simulink model "Gesamtmodell_2015b"  (R2015b)
settings: Solver=ode3  StartTime=0.0  StopTime=inf  FixedStep=dt  RelTol=1e-3
undefined symbols (not defined in the file or in its folder): Com1, dt, K1, K2, K3, Kpsi, Kx, Ky, none, sigbuilder_block, Tpsi, Tx, Ty
libraries: xpcrtudplib x9, xpcobsoletelib x4, simulink x2, xpcseriallib x1, slrtlib x1
(part 2 of 3)

== matlab function Gesamtmodell_2015b/Regelung/Robotino interface/transmit velocity, unit & direction converter ==
  settings: sampleTime=2*dtpc
  data: direction_motor0_out output; velocity_motor0_out output; direction_motor1_out output; velocity_motor1_out output; direction_motor2_out output; velocity_motor2_out output; v_x_in input; v_y_in input; v_theta_in input
%%%%%%%%%%%%%%%%%%%%%%%%%%%%%%%%%%%%%%%%%%%%%%%%%%%%%%%%%%%%%%%%%%%%%%%%%%%
% conversion from positive and/or negative longitudinal, lateral and      %
% rotational velocities (in milimeters per second) to three separate      %
% positive motor velocities (resolution: 1Byte) and their rotation        %
% direction                                                               %
%                                                                         %
% inputs:  v_x_in (longitudinal velocity in milimeters per second),       %
%          v_y_in (lateral velocity in milimeters per second),            %
%          v_theta_in (rotational velocity in milimeters per second)      %
% outputs: direction_motor0_out (rotating direction of motor0             %
%          (0 := counter-clockwise; 2 := clockwise)),                     %
%          velocity_motor0_out (from 0 to 255),                           %
%          direction_motor1_out (rotating direction of motor1             %
%          (0 := counter-clockwise; 2 := clockwise)),                     %
%          velocity_motor1_out (from 0 to 255),                           %
%          direction_motor2_out (rotating direction of motor2             %
%          (0 := counter-clockwise; 2 := clockwise)),                     %
%          velocity_motor2_out (from 0 to 255)                            %
%%%%%%%%%%%%%%%%%%%%%%%%%%%%%%%%%%%%%%%%%%%%%%%%%%%%%%%%%%%%%%%%%%%%%%%%%%%
function [direction_motor0_out, velocity_motor0_out, ...
          direction_motor1_out, velocity_motor1_out, ...
          direction_motor2_out, velocity_motor2_out] ...
                                          = fcn(v_x_in, v_y_in, v_theta_in)
%%%%%%%%%%%%%%%%%%%%%%%%%%%%%%%%%%%%%%%%%%%%%%%%%%%%%%%%%%%%%%%%%%%%%%
% conversion from longitudinal, lateral & rotational velocity to the %
% three separate motor velocities                                    %
%%%%%%%%%%%%%%%%%%%%%%%%%%%%%%%%%%%%%%%%%%%%%%%%%%%%%%%%%%%%%%%%%%%%%%
v0 = (-v_x_in * cosd(30)) + ( v_y_in * cosd(60)) + (v_theta_in * 135);
v1 =                      + (-v_y_in)            + (v_theta_in * 135);
v2 = ( v_x_in * cosd(30)) + ( v_y_in * cosd(60)) + (v_theta_in * 135);

%%%%%%%%%%%%%%%%%%%%%%%%%%%%%%%%%%%%%%%%%%%%%%%%%%%%%%%%%%%%%%%%%%%%%
% conversion of the separate motor velocities from millimeters to a %
% value between -255 and 255                                        %
%%%%%%%%%%%%%%%%%%%%%%%%%%%%%%%%%%%%%%%%%%%%%%%%%%%%%%%%%%%%%%%%%%%%%
f = 1 / 7.02;
v0 = v0 * f;
v1 = v1 * f;
v2 = v2 * f;

%%%%%%%%%%%%%%%%%%%%%%%%%%%%%%%%%%%%%%%%%%%%%%%%%%%%%%%%%%%%%%%%%%%%
% division of motor velocities into absolute velocity and rotating %
% direction                                                        %
%%%%%%%%%%%%%%%%%%%%%%%%%%%%%%%%%%%%%%%%%%%%%%%%%%%%%%%%%%%%%%%%%%%%
if v0 < 0
    direction_motor0_out =  0;
    velocity_motor0_out  = -v0;
else
    direction_motor0_out = 2;
    velocity_motor0_out  = v0;
end

if v1 < 0
    direction_motor1_out =  0;
    velocity_motor1_out  = -v1;
else
    direction_motor1_out = 2;
    velocity_motor1_out  = v1;
end

if v2 < 0
    direction_motor2_out =  0;
    velocity_motor2_out  = -v2;
else
    direction_motor2_out = 2;
    velocity_motor2_out  = v2;
end

== matlab function Gesamtmodell_2015b/Regelung/Robotino interface/serial communication/protocol adder & optional velocity adaption ==
  settings: sampleTime=2*dtpc
  data: dir input; vel input; direction_motor0_in input; velocity_motor0_in input; direction_motor1_in input; velocity_motor1_in input; direction_motor2_in input; velocity_motor2_in input; stop_in input; message output
%%%%%%%%%%%%%%%%%%%%%%%%%%%%%%%%%%%%%%%%%%%%%%%%%%%%%%%%%%%%%%%%%%%%%%%%%%%
% parameterising the 'PC104 to I/O-Board message' for serial line         %
% communication with control commands for the robotino motors             %
%                                                                         %
% optional: velocity adaption as soon as at least one motor is near the   %
%           speed limit                                                   %
%                                                                         %
% inputs: rotating directions and velocities of the three motors          %
% output: vector containing the 'PC104 to I/O-Board message' for serial   %
%         line communication                                              %
%%%%%%%%%%%%%%%%%%%%%%%%%%%%%%%%%%%%%%%%%%%%%%%%%%%%%%%%%%%%%%%%%%%%%%%%%%%
function message = fcn(dir, vel, direction_motor0_in, velocity_motor0_in, ...
                       direction_motor1_in, velocity_motor1_in, ...
                       direction_motor2_in, velocity_motor2_in, stop_in)
%%%%%%%%%%%%%%%%%%%%%%%%%%%%%%
% optional velocity adaption %
%%%%%%%%%%%%%%%%%%%%%%%%%%%%%%
vmax = 175;                                               % v_motor_dez_max

if velocity_motor0_in > vmax
    velocity_motor0_tf = velocity_motor0_in;
    
    velocity_motor0_in = vmax;
    velocity_motor1_in = vmax * velocity_motor1_in / velocity_motor0_tf;
    velocity_motor2_in = vmax * velocity_motor2_in / velocity_motor0_tf;
end

if velocity_motor1_in > vmax
    velocity_motor1_tf = velocity_motor1_in;
    
    velocity_motor0_in = vmax * velocity_motor0_in / velocity_motor1_tf;
    velocity_motor1_in = vmax;
    velocity_motor2_in = vmax * velocity_motor2_in / velocity_motor1_tf;
end

if velocity_motor2_in > vmax
    velocity_motor2_tf = velocity_motor2_in;
    
    velocity_motor0_in = vmax * velocity_motor0_in / velocity_motor2_tf;
    velocity_motor1_in = vmax * velocity_motor1_in / velocity_motor2_tf;
    velocity_motor2_in = vmax;
end
%%%%%%%%%%%%%%%%%%%%%%%%%%%%%%%%%%%%%%%%%%%%%%%%%%%%%%%%%%%%%%%%%%%%%%
% vector containing the 'PC104 to I/O-Board message' for serial line %
% communication                                                      %
%%%%%%%%%%%%%%%%%%%%%%%%%%%%%%%%%%%%%%%%%%%%%%%%%%%%%%%%%%%%%%%%%%%%%%
message = [47, abs('REC'), 5, min(stop_in), direction_motor0_in, ...
           velocity_motor0_in, zeros(1, 4), 255, 255, 255, ...
           min(stop_in), direction_motor1_in, velocity_motor1_in, ...
           zeros(1, 4), 255, 255, 255, min(stop_in), ...
           direction_motor2_in, velocity_motor2_in, zeros(1, 4), 255, ...
           255, 255, 1, dir, vel, zeros(1, 4), 255, 255, 255, abs('rec')].';

== matlab function Gesamtmodell_2015b/Regelung/Receiver/UDP interface/stop signals ==
  data: rob_number input; udp_in input; enable_out output
%%%%%%%%%%%%%%%%%%%%%%%%%%%%%%%%%%%%%%%%%%%%%%%%%%%%%%%%%%%%%%%%%%%%%%%%%%%
% Leads the enable command through. The enable command turns the Robotino %
% inputs to selectable form.                                              %
%                                                                         %
% input: udp_in (vector of 56 elements containing the data sent by the    %
%                camera-model)                                            %
% outputs: enable_out (1 = inputs are in selectable form;                 %
%                      0 = inputs are set to 0)                           %
%          udp_out (vector of 56 elements containing the data sent by the %
%                   camera-model)                                         %
%%%%%%%%%%%%%%%%%%%%%%%%%%%%%%%%%%%%%%%%%%%%%%%%%%%%%%%%%%%%%%%%%%%%%%%%%%%
function enable_out  = fcn(rob_number, udp_in)
enable_out = [0, 0];
if (udp_in(rob_number * 3 - 2) <= 0) && ...
   (udp_in(rob_number * 3 - 1) <= 0) && (udp_in(rob_number * 3) <= 0)
    enable_out(1) = 0;
else
    enable_out(1) = 1;
end
enable_out(2) = udp_in(28);

== matlab function Gesamtmodell_2015b/Regelung/Robotino interface/serial communication/error filter & protocol disassembler ==
  settings: sampleTime=dtpc/2
  data: response input; error_free_resp_in input; direction_motor0_out output; velocity_motor0_out output; direction_motor1_out output; velocity_motor1_out output; direction_motor2_out output; velocity_motor2_out output; distance_measuring_sensors_out output; di03_bump_out output; bumper_out output; error_free_resp_out output
%%%%%%%%%%%%%%%%%%%%%%%%%%%%%%%%%%%%%%%%%%%%%%%%%%%%%%%%%%%%%%%%%%%%%%%%%%%
% Error check of the 'I/O-Board to PC104 message' and filtering of this   %
% defective response: Substitute defective message by the last error free %
% message.                                                                %
% Saving of the rotating direction, velocity, shaft position and running  %
% time of the three motors. Combining all shaft positions in a vector.    %
% Combining all running times in a vector.                                %
% Saving of the three bumper bytes indicating a collision in a vector.    %
% Saving the values of the nine distance measuring IR-sensors in a vector.%
%                                                                         %
% inputs: response (actual 'I/O-Board to PC104 message')(vector 102       %
%                   elements)                                             %
%         error_free_resp_in (last error free 'I/O-Board to PC104         %
%                             message')                                   %
% outputs: directions and velocities of the three motors                  %
%          motor_positions_out (shaft positions of the three motors)      %
%                              (vector 12 elements)                       %
%          time_bytes_out (running times of the three motors)             %
%                         (vector 9 elements)                             %
%          distance_measuring_sensors_out (values of the nine IR-sensors) %
%                                         (vector 9 elements)             %
%          bumper_out (vector 3 elements)                                 %
%          error_free_resp_out (error free 'I/O-Board to PC104 message')  %
%                              (vector 102 elements)                      %
%%%%%%%%%%%%%%%%%%%%%%%%%%%%%%%%%%%%%%%%%%%%%%%%%%%%%%%%%%%%%%%%%%%%%%%%%%%
function [direction_motor0_out, velocity_motor0_out, ...
          direction_motor1_out, velocity_motor1_out, ...
          direction_motor2_out, velocity_motor2_out, ...
          distance_measuring_sensors_out, di03_bump_out, bumper_out, ...
          error_free_resp_out] = fcn(response, error_free_resp_in)
%           motor_positions_out, time_bytes_out, ...)
      
%%%%%%%%%%%%%%%%%%%%%%%%%%%%%%%%%%%%%%%%%%%%%%%%%%%%%
% filtering defective 'I/O-Board to PC104 messages' %
%%%%%%%%%%%%%%%%%%%%%%%%%%%%%%%%%%%%%%%%%%%%%%%%%%%%%
if (response(1) == 101) && (response(2) == 82) && (response(3) == 69) ...
   && (response(4) == 67) && (response(100) == 114) ...        % if the ...
   && (response(101) == 101) && (response(102) == 99)  % counter (101), ...
                        % the start (REC) and stop (rec) bytes are true ...
    error_free_resp_out = response;     % save the actual 'I/O-Board to ...
                                                           % PC104 message'
else                                                        % otherwise ...
    error_free_resp_out = error_free_resp_in;     % save the last error ...
                                        % free 'I/O-Board to PC104 message'
end

%%%%%%%%%%%%%%%%%%%%%%%%%%%%%%%%%%%%%%%%%%%%%%%%%%%%%%%%%%%%%%%%%%%%%%%%%%
% save rotating direction, velocity, shaft position and the running time %
% of motor0                                                              %
%%%%%%%%%%%%%%%%%%%%%%%%%%%%%%%%%%%%%%%%%%%%%%%%%%%%%%%%%%%%%%%%%%%%%%%%%%
direction_motor0_out  = error_free_resp_out(26);
velocity_motor0_out   = error_free_resp_out(27);
% position_motor0_byte1 = error_free_resp_out(28);
% position_motor0_byte2 = error_free_resp_out(29);
% position_motor0_byte3 = error_free_resp_out(30);
% position_motor0_byte4 = error_free_resp_out(31);
% time_motor0_byte1     = error_free_resp_out(34);
% time_motor0_byte2     = error_free_resp_out(35);
% time_motor0_byte3     = error_free_resp_out(36);

%%%%%%%%%%%%%%%%%%%%%%%%%%%%%%%%%%%%%%%%%%%%%%%%%%%%%%%%%%%%%%%%%%%%%%%%%%
% save rotating direction, velocity, shaft position and the running time %
% of motor1                                                              %
%%%%%%%%%%%%%%%%%%%%%%%%%%%%%%%%%%%%%%%%%%%%%%%%%%%%%%%%%%%%%%%%%%%%%%%%%%
direction_motor1_out  = error_free_resp_out(47);
velocity_motor1_out   = error_free_resp_out(48);
% position_motor1_byte1 = error_free_resp_out(49);
% position_motor1_byte2 = error_free_resp_out(50);
% position_motor1_byte3 = error_free_resp_out(51);
% position_motor1_byte4 = error_free_resp_out(52);
% time_motor1_byte1     = error_free_resp_out(55);
% time_motor1_byte2     = error_free_resp_out(56);
% time_motor1_byte3     = error_free_resp_out(57);

%%%%%%%%%%%%%%%%%%%%%%%%%%%%%%%%%%%%%%%%%%%%%%%%%%%%%%%%%%%%%%%%%%%%%%%%%%
% save rotating direction, velocity, shaft position and the running time %
% of motor2                                                              %
%%%%%%%%%%%%%%%%%%%%%%%%%%%%%%%%%%%%%%%%%%%%%%%%%%%%%%%%%%%%%%%%%%%%%%%%%%
direction_motor2_out  = error_free_resp_out(68);
velocity_motor2_out   = error_free_resp_out(69);
% position_motor2_byte1 = error_free_resp_out(70);
% position_motor2_byte2 = error_free_resp_out(71);
% position_motor2_byte3 = error_free_resp_out(72);
% position_motor2_byte4 = error_free_resp_out(73);
% time_motor2_byte1     = error_free_resp_out(76);
% time_motor2_byte2     = error_free_resp_out(77);
% time_motor2_byte3     = error_free_resp_out(78);

%%%%%%%%%%%%%%%%%%%%%%%%%%%%%%%%%%%%%%%%%%%
% save the three bumper bytes in a vector %
%%%%%%%%%%%%%%%%%%%%%%%%%%%%%%%%%%%%%%%%%%%
bumper_out = [error_free_resp_out(32), error_free_resp_out(53), ...
              error_free_resp_out(74)]';
          
%%%%%%%%%%%%%%%%%%%%%%%%%%%%%%%%%%%%%%%%%%%%%%%%%%%%%%%%%%%%%%%%%%%%%%
% save the values of the nine distance measuring sensors in a vector %
%%%%%%%%%%%%%%%%%%%%%%%%%%%%%%%%%%%%%%%%%%%%%%%%%%%%%%%%%%%%%%%%%%%%%%
distance_measuring_sensors_out = [error_free_resp_out(60), ...
                    error_free_resp_out(59), error_free_resp_out(44), ...
                    error_free_resp_out(39), error_free_resp_out(38), ...
                    error_free_resp_out(17), error_free_resp_out(18), ...
                    error_free_resp_out(23), error_free_resp_out(65)];
                
%%%%%%%%%%%%%%%%%%%%%%%%%%%%%%%%%%%%%%%%%%%%%%%%%%%%%%%%
% save positions of the three motor shafts in a vector %
%%%%%%%%%%%%%%%%%%%%%%%%%%%%%%%%%%%%%%%%%%%%%%%%%%%%%%%%
% motor_positions_out = [position_motor0_byte1, position_motor0_byte2, ...
%                        position_motor0_byte3, position_motor0_byte4, ...
%                        position_motor1_byte1, position_motor1_byte2, ...
%                        position_motor1_byte3, position_motor1_byte4, ...
%                        position_motor2_byte1, position_motor2_byte2, ...
%                        position_motor2_byte3, position_motor2_byte4];

%%%%%%%%%%%%%%%%%%%%%%%%%%%%%%%%%%%%%%%%%%%%%%%%%%%%%%%%%%
% save the running times of the three motors in a vector %
%%%%%%%%%%%%%%%%%%%%%%%%%%%%%%%%%%%%%%%%%%%%%%%%%%%%%%%%%%
% time_bytes_out = [time_motor0_byte1, time_motor0_byte2, ...
%                   time_motor0_byte3, time_motor1_byte1, ...
%                   time_motor1_byte2, time_motor1_byte3, ...
%                   time_motor2_byte1, time_motor2_byte2, time_motor2_byte3];

%%%%%%%%%%%%%%%%%%%%%%%%%%%%%%%%%%%%%%
% save values of digital input 0 - 3 %
%%%%%%%%%%%%%%%%%%%%%%%%%%%%%%%%%%%%%%
di03_bump_out = error_free_resp_out(32);

== matlab function Gesamtmodell_2015b/Regelung/Robotino interface/receive direction, unit & velocity converter ==
  settings: sampleTime=dtpc/2
  data: number_of_robot input; direction_motor0_in input; v_x_out output; velocity_motor0_in input; direction_motor1_in input; velocity_motor1_in input; direction_motor2_in input; velocity_motor2_in input; v_y_out output; v_theta_out output
%%%%%%%%%%%%%%%%%%%%%%%%%%%%%%%%%%%%%%%%%%%%%%%%%%%%%%%%%%%%%%%%%%%%%%%%%%%
% assembly of the three separate positive motor velocities (resolution:   %
% 1Byte) and their rotation direction to positive and/or negative         %
% longitudinal, lateral & rotational velocities (in milimeters per        %
% second)                                                                 %
%                                                                         %
% inputs:  direction_motor0_in (rotating direction of motor0              %
%          (129 := counter-clockwise; 128 := clockwise)),                 %
%          velocity_motor0_in (from 0 to 255),                            %
%          direction_motor1_in (rotating direction of motor1              %
%          (0 := counter-clockwise; 1 := clockwise)),                     %
%          velocity_motor1_in (from 0 to 255),                            %
%          direction_motor2_in (rotating direction of motor2              %
%          (0 := counter-clockwise; 1 := clockwise)),                     %
%          velocity_motor2_in (from 0 to 255)                             %
% outputs: v_x_out (longitudinal velocity (in milimeters per second)),    %
%          v_y_out (lateral velocity (in milimeters per second)),         %
%          v_theta_out (rotational velocity (in milimeters per second))   %
%%%%%%%%%%%%%%%%%%%%%%%%%%%%%%%%%%%%%%%%%%%%%%%%%%%%%%%%%%%%%%%%%%%%%%%%%%%
function [v_x_out, v_y_out, v_theta_out] ...
    = fcn(number_of_robot, direction_motor0_in, velocity_motor0_in, direction_motor1_in, ...
          velocity_motor1_in, direction_motor2_in, velocity_motor2_in)
%%%%%%%%%%%%%%%%%%%%%%%%%%%%%%%%%%%%%%%%%%%%%%%%%%%%%%%%%%%%%%%%%
% assembly of absolute motor velocity and rotating direction to %
% longitudinal, lateral & rotational velocity for every motor   %
%%%%%%%%%%%%%%%%%%%%%%%%%%%%%%%%%%%%%%%%%%%%%%%%%%%%%%%%%%%%%%%%%


% the direction bit for the motor 0 of robotino 3 is located at a different position
if number_of_robot == 3
    cmp = 1;
else
    cmp = 129;
end
    

if direction_motor0_in < cmp
    v0 = -velocity_motor0_in;
else
    v0 =  velocity_motor0_in;
end

if direction_motor1_in < 1
    v1 = -velocity_motor1_in;
else
    v1 =  velocity_motor1_in;
end

if direction_motor2_in < 1
    v2 = -velocity_motor2_in;
else
    v2 =  velocity_motor2_in;
end

%%%%%%%%%%%%%%%%%%%%%%%%%%%%%%%%%%%%%%%%%%%%%%%%%%%%%%%%%%%%%%%%%%%%%%%%%
% conversion of the separate motor velocities from a value between -255 %
% and 255 to millimeters                                                %
%%%%%%%%%%%%%%%%%%%%%%%%%%%%%%%%%%%%%%%%%%%%%%%%%%%%%%%%%%%%%%%%%%%%%%%%%
f_rcv = 7.02;
v0    = v0 * f_rcv;
v1    = v1 * f_rcv;
v2    = v2 * f_rcv;

%%%%%%%%%%%%%%%%%%%%%%%%%%%%%%%%%%%%%%%%%%%%%%%%%%%%%%%%%%%%%%%%%%%%
% conversion from three separate motor velocities to longitudinal, %
% lateral & rotational velocity                                    %
%%%%%%%%%%%%%%%%%%%%%%%%%%%%%%%%%%%%%%%%%%%%%%%%%%%%%%%%%%%%%%%%%%%%
v_x_out     = (v2 - v0) / (2 * cosd(30));                         % in mm/s
v_y_out     = (v0 - 2 * v1 + v2) / 3;                             % in mm/s
v_theta_out = (v0 + v1 + v2) / (3 * 135);                        % in rad/s

== matlab function Gesamtmodell_2015b/Regelung/Receiver/autoRobID ==
  data: udpIn input; pX output; pY output; psi output; enable output; robID input
function [pX, pY, psi, enable] = autoRobID(udpIn, robID)
enable  = 1;
pX      = 0;
pY      = 0;
psi     = 0;

if robID == 1
    pX      = udpIn(1);
    pY      = udpIn(2);
    psi     = udpIn(3);
elseif robID == 2
    pX      = udpIn(4);
    pY      = udpIn(5);
    psi     = udpIn(6);
elseif robID == 3
    pX      = udpIn(7);
    pY      = udpIn(8);
    psi     = udpIn(9);
elseif robID == 4
    pX      = udpIn(10);
    pY      = udpIn(11);
    psi     = udpIn(12);
end

if (pX == 0) && (pY == 0)
    enable = 0;
end

== matlab function Gesamtmodell_2015b/Regelung/Robotino interface/serial communication/stop by bumper ==
  settings: sampleTime=2*dtpc
  data: stop_out output; bumper input; stop_flag_in input; stop_flag_out output
%%%%%%%%%%%%%%%%%%%%%%%%%%%%%%%%%%%%%%%%%%%%%%%%%%%%%%%%%%%%%%%%%%%%%%%%%%%
% Recognition of collisions and creating of variables indicating and      %
% marking a collision                                                     %
%                                                                         %
% inputs: bumper (vector of the three bumper bytes)                       %
%         stop_flag_in (As long as no collision has occured,              %
%                       'stop_flag_in' contains the last bumper vector    %
%                       indicating no collision.                          %
%                       If a collision has occured, 'stop_flag_in'        %
%                       contains the last bumper vector indicating a      %
%                       collision until the simulation stops.)            %
% outputs: stop_out (indicates a collision: 1 = no collision;             %
%                                           0 = collision)                %
%          stop_flag_out (gets the actual bumper vector unless 'bumper'   %
%                         indicates no collision and 'stop_flag_in'       %
%                         indicates a past collision.)                    %
%%%%%%%%%%%%%%%%%%%%%%%%%%%%%%%%%%%%%%%%%%%%%%%%%%%%%%%%%%%%%%%%%%%%%%%%%%%
function [stop_out, stop_flag_out] = fcn(bumper, stop_flag_in)
if max(bumper) == 31       % as soon as the maximum value of the bumper ...
                              % vector indicates 31 a collision is detected
    stop_out = 0;
    stop_flag_out = bumper;
elseif max(stop_flag_in) == 31 % if the maximum value of 'stop_flag_in' ...
                                      % indicates a past collision (31) ...
    stop_out = 0;         % 'stop_out' gets 0 for a further stop of the ...
                                                           % motors and ...
    stop_flag_out = stop_flag_in; % 'stop_flag_out' gets the last bumper...
                                       % vector indicating a past collision
else                                                        % otherwise ...
    stop_out = 1;    % 'stop_out' gets 1 to keep the motors running and ...
    stop_flag_out = bumper; % 'stop_flag_out' gets the actual bumper vector
end

== matlab function Gesamtmodell_2015b/Regelung/Robotino interface/distance converter ==
  settings: sampleTime=dtpc/2
  data: dms_in input; dms_out output
%%%%%%%%%%%%%%%%%%%%%%%%%%%%%%%%%%%%%%%%%%%%%%%%%%%%%%%%%%%%%%%%%%%%%%%%%%%
% conversion of the nine distance measuring sensor values (resolution:    %
% 1Byte) to unit milimeters (range: from 40mm to 1500mm) with linear      %
% interpolation                                                           %
%                                                                         %
% input:  vector containing the values of the nine distance measuring     %
%         sensors                                                         %
% output: vector containing the nine values in milimeters                 %
%%%%%%%%%%%%%%%%%%%%%%%%%%%%%%%%%%%%%%%%%%%%%%%%%%%%%%%%%%%%%%%%%%%%%%%%%%%
function dms_out = fcn(dms_in)

y_mm = [40, 45, 50, 60, 75, 100, 125, 150, 175, 200, 250, 300]; % , ...
        %400, 500, 600, 700, 800, 900, 1000, 1100, 1200, 1300, 1500];
    
x_sensor = [255, 249.7733813, 228.6082474, 193.6871795, ...
            152.0044843, 113.7266187, 92.42268041, ...
            76.36407767, 65.19289827, 55.1025641, ...
            43.06299213, 34.97068404]; % , 24.37410072, ...
            % 16.3381295, 11.62589928, 8.661870504, ...
            % 6.316546763, 4.74, 3.65, 2.96, 2.40, ...
            % 2.035971223, 1.539568345];

% x_sensor = round(100 * x_sensor) / 100;

dms_out = interp1(x_sensor, y_mm, dms_in, 'linear');

== matlab function Gesamtmodell_2015b/Regelung/z(x) ==
  data: x1 input; x2 input; x3 input; x4 input; z1 output; z5 output; z2 output; z6 output; x5 input; x6 input; z3 output; z4 output
function [z1,z5,z2,z6,z3,z4]= zustandsTrafo(x1,x2,x3,x4,x5,x6)

z1 = cos(x4) * x1 - sin(x4) * x2;
z2 = sin(x4) * x1 + cos(x4) * x2;
z3 = x3;
z4 = x4;
z5 = x5;
z6 = x6;

== matlab function Gesamtmodell_2015b/Regelung/Robotino interface/light barrier & slider ==
  data: di03_bump_in input; light_barrier output; slider output
function [light_barrier, slider] = fcn(di03_bump_in)
%%%%%%%%%%%%%%%%%%%%%%%%%%%%%%%%%%%%%%%%%%%%%%%%%%%%%%%%%%%%%%%%%%%%%%%%%%%
% di03_bump_in = 0 alternatively 12 ->  no light barrier activation       %
%                                       no slider activation              %
% di03_bump_in = 13                 ->  only light barrier activation     %
% di03_bump_in = 14                 ->  only slider activation            %
% di03_bump_in = 15                 ->  light barrier activation          %
%                                       slider activation                 %
%%%%%%%%%%%%%%%%%%%%%%%%%%%%%%%%%%%%%%%%%%%%%%%%%%%%%%%%%%%%%%%%%%%%%%%%%%%
% function [light_barrier, slider] = fcn(di03_bump_in)
% bin = dec2bin(di03_bump_in);
% if bin(3) == 1
%     light_barrier = 1;
% else
%     light_barrier = 0;
% end
% if bin(4) == 1
%     slider = 1;
% else
%     slider = 0;
% end
if     di03_bump_in == 13
    light_barrier = 1;
    slider        = 0;
elseif di03_bump_in == 14
    light_barrier = 0;
    slider        = 1;
elseif di03_bump_in == 15
    light_barrier = 1;
    slider        = 1;
else
    light_barrier = 0;
    slider        = 0;
end

== stateflow chart Gesamtmodell_2015b/Regelung/Zustandsautomat/FertigunsbereichsLogik ==
  state Warten
    entry: ZielAnfordern = 1;
    exit: ZielAnfordern = 0;
  state Neue_Station_erhalten
  note: => Greifer öffnen
  note: => Warten
  state zuerst_Vorposition_anfahren
    entry: StationsNr = Ziel + 5;
  note: => Greifer schließen
  state Ziel_anfahren
    entry: StationsNr = Ziel;
  state zuerst_Vorposition_anfahren2
    entry: StationsNr = letztesZiel + 5;
  state Station_anfahren
    entry: enable = 1,
    Neue_Planung =1;
  state Station_erreicht
    entry: enable = 1,
    Neue_Planung = 0;
    exit: letztesZiel = StationsNr;
  (default) -> Warten
  Station_erreicht -> Warten [order 3] : [AktionAnZiel == 2]
      |  / {GreiferPose = 0}
  Station_erreicht -> Warten [order 4]
  Station_erreicht -> Warten [order 2] : [AktionAnZiel == 1]
      | / {GreiferPose = 1}
  Warten -> Neue_Station_erhalten : [Ziel ~= letztesZiel]
  Neue_Station_erhalten -> zuerst_Vorposition_anfahren [order 2] : [istEinFach(Ziel) &&  ...
      |  ~istVorpositionDesFachs(Ziel, letztesZiel)]
  Station_erreicht -> Neue_Station_erhalten [order 1] : [StationsNr ~= Ziel]
  Neue_Station_erhalten -> zuerst_Vorposition_anfahren2 [order 1] : [istEinFach(Ziel) &&  ...
      |  ~istVorpositionDesFachs(Ziel, letztesZiel) && istEinFach(letztesZiel)]
  Neue_Station_erhalten -> zuerst_Vorposition_anfahren2 [order 3] : [istEinFach(letztesZiel)]
  Neue_Station_erhalten -> Ziel_anfahren [order 4]
  zuerst_Vorposition_anfahren -> Station_anfahren
  Ziel_anfahren -> Station_anfahren
  zuerst_Vorposition_anfahren2 -> Station_anfahren
  Station_anfahren -> Station_erreicht : [zielPositionErreicht]
  data: ziel function_input double; antwort function_output double; Ziel function_input double; letztesZiel function_input double; antwort function_output double; Ziel input double; AktionAnZiel input double; ZielAnfordern output double =0; letztesZiel local double =0; enable output double =0; GreiferPose output double; zielPositionErreicht input; StationsNr output double =0; Neue_Planung output double
  function antwort = istEinFach(ziel):
    | function antwort = istEinFach(ziel)
    |  
    |     if 0 < mod(ziel, 10) &&  mod(ziel, 10) < 4
    |         antwort = 1;
    |     else
    |         antwort = 0;
    |     end
    | 
    | end
  function antwort = istVorpositionDesFachs(Ziel, letztesZiel):
    | function antwort = istVorpositionDesFachs(Ziel, letztesZiel)
    | 
    |     if (letztesZiel - 5) == Ziel
    |         % Fachnummer + 5 = Nummer der Vorposition
    |         antwort = 1;
    |     else
    |         antwort = 0;
    |     end
    | 
    | end

== matlab function Gesamtmodell_2015b/Regelung/Stellgrößen- beschränkung /Beschraenkung  ==
  data: MaxStellT input; MaxStellR input; x input; X output; Y output; y input; theta input; Theta output
function [X,Y,Theta] = Beschraenkung(MaxStellT,MaxStellR,x,y,theta)

if (x > MaxStellT)
    X = MaxStellT;
elseif  (x < -MaxStellT)
    X = -MaxStellT;
else 
    X = x;
end

if (y > MaxStellT)
    Y = MaxStellT;
elseif  (y < -MaxStellT)
    Y = -MaxStellT;
else
    Y = y;
end

if (theta > MaxStellR)
    Theta = MaxStellR;
elseif  (theta < -MaxStellR)
    Theta = -MaxStellR;
else
    Theta = theta;
end

== matlab function Gesamtmodell_2015b/Regelung/u(x,v)  ==
  data: v1 input; v2 input; v3 input; x1 input; x2 input; x3 input; x4 input; u1 output; u2 output; u3 output; Tx parameter; Ty parameter; Kx parameter; Ky parameter
function [u1, u2, u3]= inputLinearisierung(v1,v2,v3,x1,x2,x3,x4,Tx,Ty,Kx,Ky)


%u1 = (Ty*x1 - Tx*x1 + Ty*v1*cos(x4) + Tx*v2*sin(x4) + Tx*x1*cos(x4)^2 - Ty*x1*cos(x4)^2 - (Tx*x2*sin(2*x4))/2 + (Ty*x2*sin(2*x4))/2 + Tx*Ty*x2*x3)/Ty;
%u2 = -(Ty*x2 - Tx*x2 - Tx*v2*cos(x4) + Ty*v1*sin(x4) + Tx*x2*cos(x4)^2 - Ty*x2*cos(x4)^2 + (Tx*x1*sin(2*x4))/2 - (Ty*x1*sin(2*x4))/2 + Tx*Ty*x1*x3)/Tx;
u1 = (Ty*x1 - Tx*x1 + Tx*x1*cos(x4)^2 - Ty*x1*cos(x4)^2 - (Tx*x2*sin(2*x4))/2 + (Ty*x2*sin(2*x4))/2 + Kx*Ty*v1*cos(x4) + Ky*Tx*v2*sin(x4) + Tx*Ty*x2*x3)/(Kx*Ty);
u2 = -(Ty*x2 - Tx*x2 + Tx*x2*cos(x4)^2 - Ty*x2*cos(x4)^2 + (Tx*x1*sin(2*x4))/2 - (Ty*x1*sin(2*x4))/2 - Ky*Tx*v2*cos(x4) + Kx*Ty*v1*sin(x4) + Tx*Ty*x1*x3)/(Ky*Tx);
u3 = v3;

== matlab function Gesamtmodell_2015b/Regelung/Receiver/x4(psi) ==
  data: psi input; x4 output
function x4 = Winkelkorrektur(psi)

persistent turnCounter firstRun lastAngle

if isempty(firstRun)
    firstRun = 1;
    turnCounter = 0;
    lastAngle = 0;
end

% Kamera gibt uns -pi bis + pi
% Wir wollen 0 bis 2pi
psi = mod(psi+2*pi,2*pi);

% winkel kontinuierlich hoch bzw runterzaehlen
if( (psi < (2*pi)/5) && (lastAngle > ((2*pi) - (2*pi)/5) ) )
    turnCounter = turnCounter + 1;
end

if( (lastAngle < (2*pi)/5) && (psi > ((2*pi) - (2*pi)/5) ) )
    turnCounter = turnCounter - 1;
end

lastAngle = psi;

x4 = psi + turnCounter * 2*pi;

== matlab function Gesamtmodell_2015b/Regelung/Zustandsregler/Winkelentstoerung ==
  data: Ist input; Soll input; Out output



function Out = Winkel(Ist,Soll)

Ist = mod(Ist, 2*pi);      % Normierung des Ist-Winkels auf das Intervall 0° - 360°
Soll = mod(Soll, 2*pi);    % Normierung des Soll-Winkels auf das Intervall 0° - 360°

if (abs(Soll-Ist) <= pi)   % (1)
    
    Out = Soll - Ist;      % (2)
    
else
    
     if (Soll > Ist)                % (3)
        Out = Soll - Ist - 2*pi;    % (4)
     else
         Out = Soll - Ist + 2*pi;   % (5)
     end
end

% Problem: 
% Beim Durchschreiten der Grenze 0°/360° entsteht ein Sprung in
% der Regeldifferenz beim Winkel, der zu einer unkontrollierten Rotation
% des Robotino führt
% 
% Lösung: 
% Impelementierung einer Fallunterscheidung, die die tatsächliche
% Regeldifferenz unter Berücksichtigung der Grenze 0°/360° ausgibt
% 
% Ansatz: 
% Prüfung, ob die vorgegebene Trajektorie über die kritische Grenze
% führt (1). Führt die Trajektorie über die kritische Grenze, ist
% der Betrag der Differenz zwischen Soll- und Istwert > pi.
% 
% Bei unkritischen Trajektorien wird die Regeldifferenz über die Formel (2)
% zurückgegeben.
%
% Bei kritischen Trajektorien muss zuerst unterschieden werden, in welchem
% Drehsinn die kritische Grenze durchschritten wird (3). Bei positivem
% Drehsinn wird die Differenz nach Formel (4) ermittelt, bei negativem
% Drehsinn wird die Differenz nach Formal (5) ermittelt. 
%
% Die Ausgabe der Regeldifferenz erfolgt immer in Richtung und Betrag, bei
% einem positiven Vorzeichen befindet sich die Sollposition in mathematisch
% positivem Drehsinn, bei einem negativen Vorzeichen befindet sie sich in
% mathematisch negativem Drehsinn. Der Betrag gibt die verbleibene
% Winkeldifferenz zur Sollposition an.

== matlab function Gesamtmodell_2015b/Regelung/Zustandsautomat/KoordonatenTafel1 ==
  data: stationsNr input; zielX output; zielY output; zielPsi output; StationsKoordinaten parameter; enable output
function [zielX, zielY, zielPsi, enable] = koordinaten(stationsNr,StationsKoordinaten)

enable = 1;

% Warteposition vorne
if mod(stationsNr, 10) == 0 
    
        % WartePosition 0
        if stationsNr == 0
            %weil Matlab leider nicht von 0 aus zählen kann müssen wir das von
            %Hand abfangen...doofes Matlab
            zielX   = 853;
            zielY   = 2288;
            zielPsi = pi/2;
        else
            zielX   = StationsKoordinaten(1,stationsNr);
            zielY   = StationsKoordinaten(2,stationsNr);
            zielPsi = pi/2;
        end

% Stations-Bucht
elseif 0 < mod(stationsNr, 10) && mod(stationsNr, 10) < 4
    
    zielX   = StationsKoordinaten(1,stationsNr);
    zielY   = StationsKoordinaten(2,stationsNr);
    
    % auf welcher Seite der Station?
    if mod(stationsNr, 20) < 10
        % links
        zielPsi = 0;
    else
        % rechts
        zielPsi = pi;
    end

% Warteposition hinten
elseif mod(stationsNr, 10) == 4
    
    zielX   = StationsKoordinaten(1,stationsNr);
    zielY   = StationsKoordinaten(2,stationsNr);
    zielPsi = pi/2;

% Warteposition mitte
elseif mod(stationsNr, 10) == 5
    
    zielX   = StationsKoordinaten(1,stationsNr);
    zielY   = StationsKoordinaten(2,stationsNr);
    zielPsi = pi/2;

% Vorposition der Bucht
elseif 5 < mod(stationsNr, 10) && mod(stationsNr, 10) < 9
    
    % auf welcher Seite der Station?
    if mod(stationsNr, 20) < 10
        % links
        zielX   = StationsKoordinaten(1,stationsNr-5) - 100;
        zielY   = StationsKoordinaten(2,stationsNr-5);
        zielPsi = 0;
    else
        % rechts
        zielX   = StationsKoordinaten(1,stationsNr-5) + 100;
        zielY   = StationsKoordinaten(2,stationsNr-5);
        zielPsi = pi;
    end

% eine nicht zugeteilte Stationsnummer wird angefordert
else
    % Roboter anhalten
    enable = 0;

    zielX   = 0;
    zielY   = 0;
    zielPsi = 0;
end

== matlab function Gesamtmodell_2015b/Regelung/Zustandsautomat/zielErreicht ==
  data: roboX input; erreicht output; roboY input; roboPsi input; zielX input; zielY input; zielPsi input
function erreicht = zielErreicht(roboX, roboY, roboPsi, zielX, zielY, zielPsi)

    transToleranz = 5;
    rotToleranz = pi/10;

    erreicht = 0;
    
    if( abs(zielX-roboX) > transToleranz)
        return;
    end 
    
    if( abs(zielY-roboY) > transToleranz)
        return;
    end 
       
    if( abs(zielPsi-roboPsi) > rotToleranz)
        return;
    end   

    erreicht = 1;

end

== matlab function Gesamtmodell_2015b/Regelung/Kalman ==
  data: vxZustand input; vyZustand input; vPsiZustand input; PsiZustand input; xZustand input; yZustand input; enable input; dt parameter; vx output; vy output; vpsi output; pospsi output; posx output; posy output; Tx parameter; Ty parameter; Tpsi parameter; Kx parameter; Ky parameter; Kpsi parameter; enableBeob output
function [vx,vy,vpsi,pospsi,posx,posy,enableBeob] = fcn(vxZustand,vyZustand,vPsiZustand,PsiZustand,xZustand,yZustand,enable,dt,Tx,Ty,Tpsi,Kx,Ky,Kpsi)

persistent A H Q R 
persistent x P
persistent firstRun found
QVel = 0.01; 
QPos = 0.01;
if isempty(firstRun)
found = 0;
x = [0; 0; 0; 0; 2000; 1600];
    

A= [1       0       0       0       0       0;
    0       1       0       0       0       0;
    0       0       1       0       0       0;
    0       0       dt      1       0       0;
    dt      0       0       0       1       0;
    0       dt      0       0       0       1];
    
H = [0 0 0 1 0 0;
     0 0 0 0 1 0;
     0 0 0 0 0 1];

Q = [QVel       0       0       0       0       0;
     0       QVel       0       0       0       0;
     0          0       QVel    0       0       0;
     0          0       0       QPos    0       0;
     0          0       0       0       QPos    0;
     0          0       0       0       0    QPos];
   
  R = 1;

  P =  [1       0       0       0       0       0;
        0       1       0       0       0       0;
        0       0       1       0       0       0;
        0       0       0       1000       0       0;
        0       0       0       0       1000       0;
        0       0       0       0       0       1000];
  
  firstRun = 1;  
end


x =[vxZustand ; vyZustand; vPsiZustand; PsiZustand;x(5:end,1)];

x = A*x;  
P = A*P*A' + Q;    
dist = 0;
Rnow = R;
if enable == 1
    z = [PsiZustand;xZustand;yZustand];
    % Reduzierung der Glaubwürdigkeit bei weit entfernten Messungen
    dist = sqrt(abs(z(2)-x(5))^2 + abs(z(3)-x(6))^2);

    if (PsiZustand == 0 && xZustand == 0 && yZustand == 0)
        Rnow = 1000000000;
    elseif dist > 20
        Rnow = 0;
        found = 0;
    elseif dist < 20
        found =1;
        Rnow = 0;
    else 
        Rnow = R;
    end
    
    K =    P*H'*inv(H*P*H' + Rnow*eye(3)); 

    x = x + K*(z - H*x);

    P = P - K*H*P;
end
enableBeob = found;

vx      = x(1);
vy      = x(2);
vpsi    = x(3);
pospsi  = x(4);
posx    = x(5);
posy    = x(6);

== matlab function Gesamtmodell_2015b/Regelung/enable  ==
  data: enable1 input; enable output; enable2 input; enable3 input; enable4 input; enable5 input
function enable  = enable(enable1,enable2,enable3,enable4,enable5)
    if enable1 && (enable2 || enable4 )&& enable3 && enable5
        enable = 1;
    else 
        enable = 0;
    end
end

== matlab function Gesamtmodell_2015b/Regelung/Zustandsautomat/positionsPlanung ==
  data: neuePlanung input; zielPsi input; zielY input; xSoll output; zielX input; psiIst input; yIst input; xIst input; ySoll output; psiSoll output; dt parameter
function [xSoll, ySoll, psiSoll] = positionsPlanung(neuePlanung,zielPsi, zielY, zielX, psiIst,yIst,xIst,dt)
    vXSoll      = 100;
    vYSoll      = 100;
    vPsiSoll    = 0.5;
    transToleranz = 10;
    rotToleranz = pi/10;
    
    persistent n lastNeuePlanung startX startY startPsi x_SollOld y_SollOld psi_SollOld tryAgain firstRun 
    
    if isempty(firstRun)
        firstRun    = 1;
        n           = 0;
        lastNeuePlanung  = 0;
        tryAgain    = 0;
        startX      = xIst;
        startY      = yIst;
        startPsi    = psiIst;
        x_SollOld   = xIst;
        y_SollOld   = yIst;
        psi_SollOld = psiIst;
    end
    
    if (neuePlanung == 1 && lastNeuePlanung == 0) || tryAgain
        if (xIst == 0) || (yIst == 0)
            tryAgain = 1;
        else 
            startX      = xIst;
            startY      = yIst;
            startPsi    = psiIst;
            x_SollOld   = xIst;
            y_SollOld   = yIst;
            psi_SollOld = psiIst;
            tryAgain = 0;
        end
    end
    
    lastNeuePlanung = neuePlanung;  
    
    if (neuePlanung == 1) && (tryAgain == 0) 
        if(abs(zielX - xIst) > transToleranz) && (zielX > xIst) 
            %x_Soll      = vXSoll   * n * dt + startX;
            xSoll = x_SollOld + vXSoll * dt;
        elseif (abs(zielX - xIst) > transToleranz) && (zielX < xIst)
            %x_Soll      = - vXSoll   * n * dt + startX;
            xSoll = x_SollOld - vXSoll * dt;
        else
            xSoll      = zielX;
        end 
        
        if( abs(zielY-yIst) > transToleranz) && (zielY > yIst)
            %y_Soll      = vYSoll   * n * dt + startY;
            ySoll = y_SollOld + vYSoll * dt;
        elseif (abs(zielY - yIst) > transToleranz) && (zielY < yIst)
            %y_Soll      = - vYSoll   * n * dt + startY;  
            ySoll = y_SollOld - vYSoll * dt;
        else
            ySoll      = zielY;
        end 

        if( abs(zielPsi-psiIst) > rotToleranz) && (zielPsi > psiIst)
            %psi_Soll    = vPsiSoll * n * dt + startPsi;
            psiSoll = psi_SollOld + vPsiSoll * dt;
        elseif (abs(zielPsi - psiIst) > rotToleranz) && (zielPsi < psiIst)
            %psi_Soll    = - vPsiSoll * n * dt + startPsi;
            psiSoll = psi_SollOld - vPsiSoll * dt;
        else
            psiSoll    = zielPsi;
        end  
        x_SollOld = xSoll;
        y_SollOld = ySoll;
        psi_SollOld = psiSoll;
        n = n + 1;
    else
        xSoll      = xIst;
        ySoll      = yIst;
        psiSoll    = psiIst;
        n = 0;
    end
    
end

== matlab function Gesamtmodell_2015b/Regelung/NewCam ==
  data: yZustand input; xZustand input; psiZustand input; enable output
function enable = fcn(yZustand,xZustand,psiZustand)


persistent oldx oldy oldpsi firstRun

if isempty(firstRun)
   firstRun = 1;
   oldx     = -1;
   oldy     = -1;
   oldpsi   = -1;
end
firstRun = firstRun +1;
if firstRun < 2
    firstRun = firstRun +1;
    enable =0;
else  
    if((mod(firstRun,1) == 0)&&((oldx ~= xZustand) || (oldy ~= yZustand) || (oldpsi ~= psiZustand)))
        enable = 1;
       oldx     = xZustand;
       oldy     = yZustand;
       oldpsi   = psiZustand;

    else
        enable = 0;
    end
end

== matlab function Gesamtmodell_2015b/Regelung/Bereichswaehler ==
  data: modus output; transportbereich input; enable output; fertigungsbereich input
function [modus, enable] = fcn(transportbereich, fertigungsbereich)

enable = false;
modus = 0;

if fertigungsbereich == 1 && transportbereich == 0
    enable = true;
    modus = 1;
end
    
if fertigungsbereich == 0 && transportbereich == 1
    enable = true;
    modus = 0;
end

== stateflow chart Gesamtmodell_2015b/Bahnplanung/Auftrags_Koordination ==
  settings: updateMethod=DISCRETE  sampleTime=0.02
  state Auftragskoordination
    state WerkstueckAufgenommen
      entry:Werkstueck=1,
      AktuellesZiel=ZielPos;
    state KeinWerkstueckAufgenommen
      entry:Werkstueck=0,
      AktuellesZiel=WerkstueckPos;
    state AufAuftragWarten
      entry:Werkstueck=0,
      AktuellesZiel=100;
    KeinWerkstueckAufgenommen -> WerkstueckAufgenommen : [Werkstueckerkannt==1 && Transportbereich==1]
    WerkstueckAufgenommen -> AufAuftragWarten : [Werkstueckerkannt==0 && Transportbereich==1]
    AufAuftragWarten -> KeinWerkstueckAufgenommen : [NeuerAuftrag]
    (default) -> AufAuftragWarten
  data: NeuerAuftrag input; WerkstueckPos input; ZielPos input; AktuellesZiel output; Werkstueck output; Werkstueckerkannt input; Transportbereich input

== stateflow chart Gesamtmodell_2015b/Bahnplanung/Fifo Steuerung/Fifo ==
  settings: updateMethod=DISCRETE  sampleTime=0.02
  state FIFOStationen
    state Auftrag_Roboter_1
    state Zielbereich_untersuchen
      entry:
      ersterFifo=floor(Zielstation/2)*3+2*mod(Zielstation,2)+1;
    state Fifo_einfachbesetzt1
      entry:
      zweiterFifo=floor(Zielstation/2)*3+1+1;
      Fifo=2;
    state Fifo_frei
      entry:
      Fifo=1;
    state Fifo_doppelt_besetzt
      entry:
      dritterFifo=floor(Zielstation/2)*3+2-2*mod(Zielstation,2)+1;
      Fifo=3;
    state Fifo_voll
      entry:
      Fifo=4;
    state Uebergabepunkt_gleich_Zielpunkt
      entry:
      Fifo=0;
    (default) -> Auftrag_Roboter_1
    Auftrag_Roboter_1 -> Zielbereich_untersuchen : [Zielposition>-1]
    Zielbereich_untersuchen -> Fifo_einfachbesetzt1 [order 1] : [(FifoArray(ersterFifo)~=0)| (FifoArray(ersterFifo)==0 & StationArray(Zielstation+1)~=0) ]
    Uebergabepunkt_gleich_Zielpunkt -> Zielbereich_untersuchen
    Zielbereich_untersuchen -> Uebergabepunkt_gleich_Zielpunkt [order 2]
    Fifo_einfachbesetzt1 -> Fifo_frei [order 2] : [FifoArray(ersterFifo)==0]
    Fifo_einfachbesetzt1 -> Fifo_doppelt_besetzt [order 1] : [(FifoArray(zweiterFifo)~=0)]
    Fifo_doppelt_besetzt -> Fifo_voll [order 2] : [(FifoArray(dritterFifo)~=0)]
    Fifo_frei -> Uebergabepunkt_gleich_Zielpunkt : [ StationArray(Zielstation+1)==0]
    Fifo_doppelt_besetzt -> Fifo_einfachbesetzt1 [order 1] : [FifoArray(zweiterFifo)==0]
    Fifo_voll -> Fifo_doppelt_besetzt : [FifoArray(dritterFifo)==0]
  state Wartebereich
    entry: Fifo=4;
  state Ladestation
    entry: Fifo=0;
  (default) -> Wartebereich
  Wartebereich -> FIFOStationen [order 1] : [Zielstation<8]
  FIFOStationen -> Wartebereich [order 1] : [Zielstation==10]
  Ladestation -> Wartebereich [order 1] : [Zielstation==10]
  Wartebereich -> Ladestation [order 2] : [Zielstation>=8 & Zielstation<10]
  Ladestation -> FIFOStationen [order 2] : [Zielstation<8]
  FIFOStationen -> Ladestation [order 2] : [Zielstation>=8 & Zielstation<10]
  data: FifoArray input; Zielposition input; Zielstation input; Fifo output; StationArray input; dritterFifo local; zweiterFifo local; ersterFifo local

== matlab function Gesamtmodell_2015b/Bahnplanung/Fifo Steuerung/Globale Markierung ==
  data: Robbi input; FifoArray input; FifoArray1 output; StationArray1 output; LadeArray input; LadeArray1 output
function [FifoArray1,StationArray1,LadeArray1]= fcn(Robbi,FifoArray,LadeArray)
X=zeros([1 4]);
Y=zeros([1 4]);
X=[Robbi(1) Robbi(4) Robbi(7) Robbi(10)];
Y=[Robbi(2) Robbi(5) Robbi(8) Robbi(11)];
FifoArray1=zeros([1 12]);
FifoArray1=FifoArray(1:12);
StationArray1=zeros([1 8]);
LadeArray1=zeros([1 2]);
LadeArray1=LadeArray(1:2);
N=zeros([1 4]);
S=zeros([1 4]);
L=zeros([1 4]);
for n= 1 : 1 : 4
    L(n)=round((Y(n)-2592)/500)+1;
    N(n)=round((X(n)-703)/400)+1;   % Berechnung in welchem Fifo der Roboter sich befindet
    S(n)=round((X(n)-900)/560)+1;   %Berechnung in welcher Station der Roboter sich befindet
     if (X(n)<=6000 || X(n)>6500)
        for i=1:2
            if LadeArray1(i)==n
                LadeArray1(i)=0;
            end
        end
     end
    if (X(n)>6000 && X(n)<=6500 && Y(n)>2300 && Y(n)<=3300)
        LadeArray1(L(n))=n;
    end  
   
    for i=1:8
          if StationArray1(i)==n
                StationArray1(i)=0;
          end
    end
    if (Y(n)>2100 && Y(n)<3300 && X(n)<5100) && S(n)<=8
         for i=1:12
            if FifoArray1(i)==n
                FifoArray1(i)=0;
            end
         end
       
        StationArray1(S(n))=n;
        
    elseif (Y(n)<450 && (X(n)>100 && X(n)<5250))
        for i=1:12
            if FifoArray1(i)==n
                FifoArray1(i)=0;
            end
        end
            FifoArray1(N(n))=n;
           
    elseif (X(n)>6000)
        for i=1:12
            if FifoArray1(i)==n
                FifoArray1(i)=0;
            end
        end
            FifoArray1(N(n))=n;
    end
    end
end

== matlab function Gesamtmodell_2015b/Bahnplanung/Fifo Steuerung/Positionszuweisung ==
  data: Fifo input; Zielstation input; Endposition output; RoboterID input
function Endposition = fcn(Fifo,Zielstation,RoboterID)
Endposition=zeros([1 2]);

WartepositionX= 6311;
WartepositionY=[550 950 1350 1750 2150];

StationvorneX=[853 1361 2058 2559 3256 3762 4448 4953 6311 6311];
StationvorneY=[2300 2300 2300 2300 2300 2300 2300 2300 2592 3080];
%Stationhinten=[856 1364 2059 2560 3259 3763 4451 4958];

ersterFifo=floor(Zielstation/2)*3+2*mod(Zielstation,2);
zweiterFifo=floor(Zielstation/2)*3+1;
dritterFifo=floor(Zielstation/2)*3+2-2*mod(Zielstation,2);

if Fifo==0
    Endposition(1)=StationvorneX(Zielstation+1);
    Endposition(2)=StationvorneY(Zielstation+1);
    else if Fifo==1
        Endposition(1)= ersterFifo*400+703;
        Endposition(2)= 250;
       
    else if Fifo==2
            Endposition(1)= zweiterFifo*400+703;
            Endposition(2)= 250;
        
    else if Fifo==3
            Endposition(1)= dritterFifo*400+703;
            Endposition(2)= 250;
            else
            Endposition(2)= WartepositionY(RoboterID);
            Endposition(1)= WartepositionX;
        end
        end
        end
end
end

== matlab function Gesamtmodell_2015b/Bahnplanung/Fifo Steuerung/ZielPosSplitten ==
  data: AktuellesZiel input; ZielPos output; Zielstation output
function [ZielPos,Zielstation]= fcn(AktuellesZiel)
ZielPos=mod(AktuellesZiel,10);
Zielstation=round(AktuellesZiel/10);

== matlab function Gesamtmodell_2015b/Bahnplanung/Fifo Steuerung/ZielStation_Erreicht ==
  data: Zielstation input; Erreicht output; AktuellePos input; Zielpos input
function Erreicht = fcn(Zielstation , AktuellePos,Zielpos)
X=AktuellePos(1);
Y=AktuellePos(2);
Abstand=sqrt((X-Zielpos(1))^2+(Y-Zielpos(2))^2);
%S=round((X-900)/560);
if Y >2000 && Y<2500&& X>600 && X < 5200 && Abstand<100
    Erreicht=1;
else
    Erreicht=0;
end
